simulink model "CASE_i_12a"  (R2020a)
settings: Solver=ode45  StartTime=0.0  StopTime=60  RelTol=1e-3  EnableMultiTasking=on
libraries: simulink x1
settings Model: Creator=Prof Francisco M. Gonzalez-Longatt  LastModifiedBy=fglon
settings DataIOCC: LimitDataPoints=on  SaveFormat=Array  SignalLoggingSaveFormat=ModelDataLogs  ReturnWorkspaceOutputs=off  SignalLoggingName=sigsOut
settings OptimizationCC: ExpressionDepthLimit=2147483647  LifeSpan=inf
settings DebuggingCC: SaveWithParameterizedLinksMsg=none  UnderspecifiedInitializationDetection=Classic  MergeDetectMultiDrivingBlocksExec=none  SignalResolutionControl=TryResolveAllWithWarning  MultiTaskDSMMsg=warning  MultiTaskCondExecSysMsg=none  FcnCallInpInsideContextMsg=warning  StateNameClashWarn=warning  SFUnexpectedBacktrackingDiag=warning  SFNoUnconditionalDefaultTransitionDiag=warning  SFExecutionAtInitializationDiag=none  ArithmeticOperatorsInVariantConditions=warning
settings HardwareCC: ProdBitPerPointer=32  ProdBitPerSizeT=32  ProdBitPerPtrDiffT=32  ProdLargestAtomicFloat=None  ProdIntDivRoundTo=Undefined  ProdEndianess=Unspecified  ProdWordSize=32  ProdHWDeviceType=32-bit Generic  TargetUnknown=on
settings ModelReferenceCC: PropagateSignalLabelsOutOfModel=off
settings SFSimCC: SimUseLocalCustomCode=off  CustomCodeUndefinedFunction=UseInterfaceOnly
settings RTWCC: RTWUseLocalCustomCode=off
settings CodeAppCC: StateflowObjectComments=on
settings GRTTargetCC: TargetLangStandard=C89/C90 (ANSI)  CombineOutputUpdateFcns=off  GRTInterface=on
settings ConfigComp: CovMetricSettings=dw  CovHtmlReporting=on  CovSaveCumulativeToWorkspaceVar=on  CovSaveSingleToWorkspaceVar=on  CovExternalEMLEnable=off

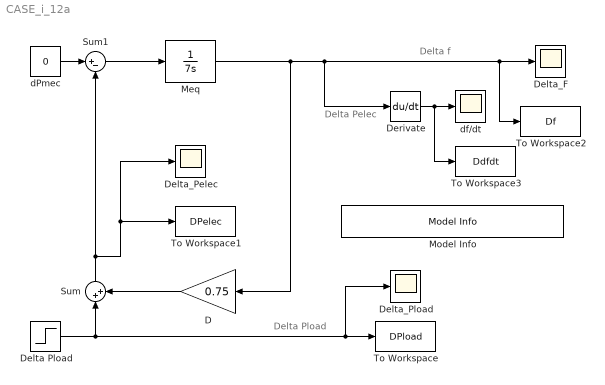
== system CASE_i_12a ==
  note: Delta Pelec
  note: Delta Pload
  note: Delta f
  D : Gain  Gain=0.75  SaturateOnIntegerOverflow=on  OutDataTypeStr=Inherit: Same as input  ParamDataTypeStr=Inherit: Same as input
  Delta Pload : Step  Time=0  After=+0.05  SampleTime=0
  Delta_F : Scope
  Delta_Pelec : Scope
  Delta_Pload : Scope
  Derivate : Derivative
  Meq : TransferFcn  Denominator=[7 0]
  Model Info : simulink/Model-Wide Utilities/Model Info  Frame=on  DisplayStringWithTags=|  HorizontalTextAlignment=Center  LeftAlignmentValue=0.5
      | Rotating Mass Model
      | %<Creator>
  Sum : Sum  Inputs=|++  SaturateOnIntegerOverflow=on
  Sum1 : Sum  Inputs=|+-  SaturateOnIntegerOverflow=on
  To Workspace : ToWorkspace  VariableName=DPload  SampleTime=-1
  To Workspace1 : ToWorkspace  VariableName=DPelec  SampleTime=-1
  To Workspace2 : ToWorkspace  VariableName=Df  SampleTime=-1
  To Workspace3 : ToWorkspace  VariableName=Ddfdt  SampleTime=-1
  dPmec : Constant  Value=0
  df/dt : Scope
  wires:
  Meq/1 -> D/1, Delta_F/1, To Workspace2/1, Derivate/1
  D/1 -> Sum/2
  Delta Pload/1 -> Sum/1, To Workspace/1, Delta_Pload/1
  Sum1/1 -> Meq/1
  Sum/1 -> Sum1/2, To Workspace1/1, Delta_Pelec/1
  dPmec/1 -> Sum1/1
  Derivate/1 -> To Workspace3/1, df/dt/1
